simulink model "SMC_asintotico_seg_tray"  (R2026b)
settings: Solver=ode4  StopTime=40  FixedStep=0.0001
settings Model: Creator=nestorhernandezcastellanos  LastModifiedBy=nestorhernandezcastellanos

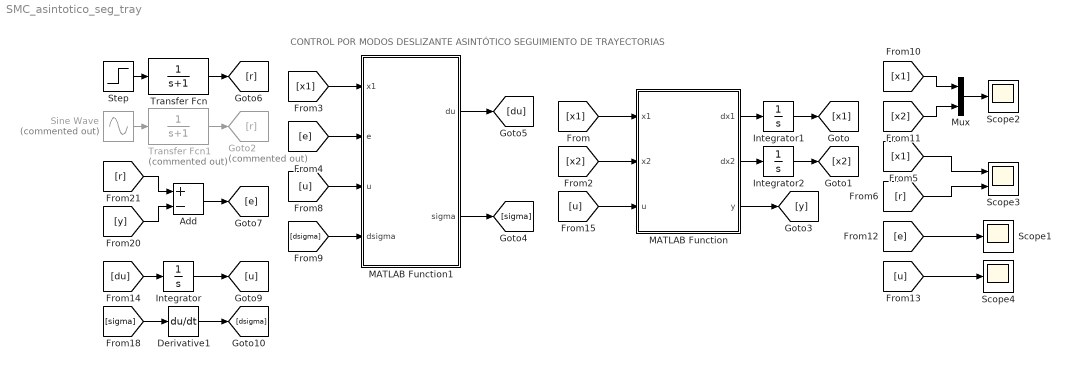
== system SMC_asintotico_seg_tray ==
  note: CONTROL POR MODOS DESLIZANTE ASINTÓTICO SEGUIMIENTO DE TRAYECTORIAS
  Add : Sum  Inputs=+-
  Derivative1 : Derivative
  Goto2 : Goto  Commented=on  GotoTag=r
  Integrator : Integrator
  Integrator1 : Integrator  InitialCondition=0.5
  Integrator2 : Integrator  InitialCondition=-5
  MATLAB Function : MATLAB Function  TreatAsAtomicUnit=on
  MATLAB Function1 : MATLAB Function  TreatAsAtomicUnit=on
  Mux : Mux  Inputs=2
  Scope1 : Scope
      settings: ActiveDisplayYMinimum=-1.8973615582703429  ActiveDisplayYMaximum=1.9955121080178562
  Scope2 : Scope
      settings: ActiveDisplayYMinimum=-6.8835029858188888  ActiveDisplayYMaximum=6.6676277959512644  DataLoggingVariableName=ScopeData2
  Scope3 : Scope  NumInputPorts=2
      settings: ActiveDisplayYMinimum=-3.0131805633261095  ActiveDisplayYMaximum=6.1417057742892585  DataLoggingVariableName=ScopeData3
  Scope4 : Scope
      settings: ActiveDisplayYMinimum=-13.087303078559547  ActiveDisplayYMaximum=13.535787080239297
  Sine Wave : Sin  Commented=on  SampleTime=0
  Step : Step  Time=10  FinalValue=5  SampleTime=0
  Transfer Fcn : TransferFcn  Denominator=[1 1]
  Transfer Fcn1 : TransferFcn  Commented=on  Denominator=[1 1]
  wires:
  MATLAB Function1/1(du) -> [du]
  MATLAB Function/2(dx2) -> Integrator2/1
  MATLAB Function/1(dx1) -> Integrator1/1
  Mux/1 -> Scope2/1
  [x1] -> MATLAB Function/1(x1)
  [x2] -> MATLAB Function/2(x2)
  [x1] -> MATLAB Function1/1(x1)
  [e] -> MATLAB Function1/2(e)
  [x1] -> Scope3/1
  [r] -> Scope3/2
  Integrator2/1 -> [x2]
  Integrator1/1 -> [x1]
  MATLAB Function/3(y) -> [y]
  [x2] -> Mux/2
  [x1] -> Mux/1
  [e] -> Scope1/1
  [u] -> Scope4/1
  Derivative1/1 -> [dsigma]
  [sigma] -> Derivative1/1
  Integrator/1 -> [u]
  [du] -> Integrator/1
  [u] -> MATLAB Function1/3(u)
  [dsigma] -> MATLAB Function1/4(dsigma)
  MATLAB Function1/2(sigma) -> [sigma]
  [u] -> MATLAB Function/3(u)
  [r] -> Add/1
  [y] -> Add/2
  Add/1 -> [e]
  Step/1 -> Transfer Fcn/1
  Transfer Fcn/1 -> [r]
  Sine Wave/1 -> Transfer Fcn1/1
  Transfer Fcn1/1 -> Goto2/1

== matlab function SMC_asintotico_seg_tray/MATLAB Function1 ==
  data: x1 input; e input; u input; du output; dsigma input; sigma output
function [du, sigma]= controlador(x1, e, u, dsigma)

% Ganancia K>1
K = 115;

% Valor arbitrario positivo
m = 4.57;
ms = 72;

sigma = e + m*x1;
s = dsigma + ms*sigma;
du = +m*ms*e - (m+ms)*u - K*sign(s);

== matlab function SMC_asintotico_seg_tray/MATLAB Function ==
  data: x1 input; x2 input; dx1 output; u input; dx2 output; y output
function [dx1, dx2, y] = planta(x1, x2, u)

dx1 = x2;
dx2 = sin(x1+x2) + cos(x1*x2) + u;

y = x1;
